simulink model "motors"  (R2017a)
settings: Solver=VariableStepAuto  StartTime=0.0  StopTime=10.0  RelTol=1e-3
PreLoadFcn:
  | pid_tester
values from neighbouring files (symbols this model uses):
  b = 0.1    [motor_params.m]
  J = 0.01    [motor_params.m]
  K = 0.01    [motor_params.m]
  L = 0.5    [motor_params.m]
  R = 1    [motor_params.m]
libraries: simulink x1
settings Model: Creator=mini  LastModifiedBy=callmetim

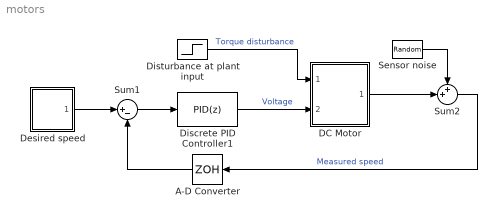
== system motors ==
  " Disturbance at plant input" : Step  Time=5  After=0.2  SampleTime=0
  A-D Converter : ZeroOrderHold  SampleTime=0.02
  DC Motor : Subsystem  mask(DC Motor){b=b, J=J, K=K, R=R, L=L}
      mask prompts: b "Damping:"; J "Inertia:"; K "Back EMF:"; R "Resistance:"; L "Inductance:"
      mask help: An ideal model of a DC Motor
      mask Help: This is <b>more elaborate<b> help.
      mask Display:
      | img = strcat(motorsPath, 'dcmotor.jpg');
      | image(imread(img));
  Desired speed : Subsystem
  Discrete PID Controller1 : simulink/Continuous/PID Controller  Controller=PID  TimeDomain=Discrete-time  SampleTime=0.02  IntegratorMethod=Forward Euler  FilterMethod=Forward Euler  Form=Parallel  UseFilter=on  ControllerParametersSource=internal  P=17.9947607768602  I=41.8923134387203  D=-0.685067684451754  N=3.3394404818866  InitialConditionSource=internal  InitialConditionForIntegrator=0  InitialConditionForFilter=0  ExternalReset=none  LimitOutput=off  UpperSaturationLimit=10  LowerSaturationLimit=-10  LinearizeAsGain=on  AntiWindupMode=back-calculation  Kb=1  TrackingMode=off  Kt=1  PParamMin=[]  PParamMax=[]  IParamMin=[]  IParamMax=[]  DParamMin=[]  DParamMax=[]  NParamMin=[]  NParamMax=[]  KbParamMin=[]  KbParamMax=[]  KtParamMin=[]  KtParamMax=[]  POutMin=[]  POutMax=[]  IOutMin=[]  IOutMax=[]  DOutMin=[]  DOutMax=[]  NOutMin=[]  NOutMax=[]  KbOutMin=[]  KbOutMax=[]  KtOutMin=[]  KtOutMax=[]  IntegratorOutMin=[]  IntegratorOutMax=[]  FilterOutMin=[]  FilterOutMax=[]  SumOutMin=[]  SumOutMax=[]  SumI1OutMin=[]  SumI1OutMax=[]  SumI2OutMin=[]  SumI2OutMax=[]  SumI3OutMin=[]  SumI3OutMax=[]  SumDOutMin=[]  SumDOutMax=[]  SaturationOutMin=[]  SaturationOutMax=[]  IntegratorContinuousStateAttributes=''  IntegratorStateMustResolveToSignalObject=off  IntegratorRTWStateStorageClass=Auto  FilterContinuousStateAttributes=''  FilterStateMustResolveToSignalObject=off  FilterRTWStateStorageClass=Auto  DifferentiatorICPrevScaledInput=0  DifferentiatorOutMin=[]  DifferentiatorOutMax=[]  InitialConditionSetting=State (most efficient)
  Sensor noise : RandomNumber  Variance=0.05  SampleTime=0
  Sum1 : Sum  Inputs=|+-
  Sum2 : Sum  Inputs=++|
  wires:
  Sum2/1 -> A-D Converter/1  "Measured speed"
  Sensor noise/1 -> Sum2/1
  Sum1/1 -> Discrete PID Controller1/1
  Discrete PID Controller1/1 -> DC Motor/2(Voltage)  "Voltage"
  DC Motor/1(Speed) -> Sum2/2
  " Disturbance at plant input"/1 -> DC Motor/1(Torque)  "Torque disturbance"
  Desired speed/1(Speed) -> Sum1/1
  A-D Converter/1 -> Sum1/2

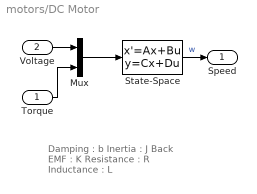
== system motors/DC Motor ==
  note: Damping : b
      | Inertia : J
      | Back EMF : K
      | Resistance : R
      | Inductance : L
  Torque : Inport
  Voltage : Inport  Port=2
  Mux : Mux  Inputs=2
  State-Space : StateSpace  A=[-b/J K/J; -K/L -R/L]  B=[0 -1/J; 1/L 0]  C=[1 0]  D=[0 0]  X0=0
  Speed : Outport
  wires:
  Mux/1 -> State-Space/1
  Voltage/1 -> Mux/1
  State-Space/1 -> Speed/1  "w"
  Torque/1 -> Mux/2

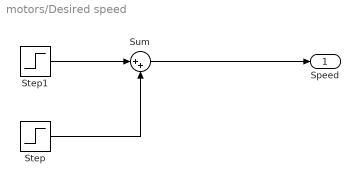
== system motors/Desired speed ==
  Step : Step  Time=7  After=-4  SampleTime=0.02
  Step1 : Step  After=2  SampleTime=0.02
  Sum : Sum  Inputs=|++
  Speed : Outport
  wires:
  Step/1 -> Sum/2
  Step1/1 -> Sum/1
  Sum/1 -> Speed/1
